simulink model "a2e1a"  (R2020a)
settings: Solver=VariableStepAuto  StartTime=0.0  StopTime=40.0  RelTol=1e-3
settings Model: Creator=mumun  LastModifiedBy=mumun

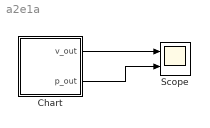
== system a2e1a ==
  Chart : Stateflow chart  TreatAsAtomicUnit=on
  Scope : Scope  NumInputPorts=2
  wires:
  Chart/2(p_out) -> Scope/2
  Chart/1(v_out) -> Scope/1

== stateflow chart a2e1a/Chart ==
  settings: updateMethod=CONTINUOUS  executeAtInitialization=1
  state Falling
    du:
    p_dot = v;
    v_dot = 0;
    p_out = p;
    v_out = v;
  (default) -> Falling : {initialize();}
  Falling -> Falling : [boundarycrossing()]{resetposition()}
  data: yn function_output double; v local double size=[1 2]; v_out output double size=[1 2]; p_out output double size=[1 2]; tableLen local double; tableWid local double; p local double size=[1 2]; holesize local double
  data v settings: updateMethod=SF_CONTINUOUS_TIME_DATA
  data p settings: updateMethod=SF_CONTINUOUS_TIME_DATA
  function initialize:
    | function initialize
    | 
    | p = [1 2]; %initial position of the ball in the board 
    | v = [1 1]; %initial velocity of the ball in x-y direction
    | tableLen= 2; %length of the table
    | tableWid= 1; %width of the table
    | 
    | 
    | end
  function resetposition:
    | function resetposition
    | 
    | if p(1,1) < 0
    |     p(1,1) = -p(1,1);
    |     v(1,1) = -1*v(1,1);
    |     v(1,2) = 1*v(1,2);
    | elseif p(1,1) > tableLen
    |     p(1,1) = 2*tableLen-p(1,1);
    |     v(1,1) = -1*v(1,1);
    |     v(1,2) = 1*v(1,2);
    | end
    | if p(1,2) < 0
    |     p(1,2) = -p(1,2);
    |     v(1,2) = -1*v(1,2);
    |     v(1,1) = 1*v(1,1);
    | elseif p(1,2) > tableWid
    |     p(1,2) = 2*tableWid-p(1,2);
    |     v(1,2) = -1*v(1,2);
    |     v(1,1) = 1*v(1,1);
    |    
    | end
  function yn = boundarycrossing:
    | function yn = boundarycrossing
    | 
    | if  p(1,1) < 0 || p(1,1) > tableLen || ...
    |     p(1,2) < 0 || p(1,2) > tableWid
    |     
    |     yn = 1;
    |     return;
    | end      
    | yn = 0;
